simulink model "mstruct_bus1"  (Simulink 6.3)
settings: Solver=ode5  StartTime=0.0  StopTime=30  RelTol=1e-3
PreLoadFcn:
  | load mstruct_bus1_data
settings Model: Creator=The MathWorks Inc.  LastModifiedBy=mshakeri  ExtModeAutoUpdateStatusClock=off  StrictBusMsg=ErrorLevel1
settings DataIOCC: SignalLoggingName=logsOut
settings OptimizationCC: InlineParams=on  InlineInvariantSignals=on
settings DebuggingCC: CheckExecutionContextPreStartOutputMsg=on  CheckExecutionContextRuntimeOutputMsg=on  SolverPrmCheckMsg=none
settings HardwareCC: TargetHWDeviceType=32-bit Generic
settings ModelReferenceCC: UpdateModelReferenceTargets=IfOutOfDate
settings RTWCC: ProcessScript=grt_make_rtw_hook

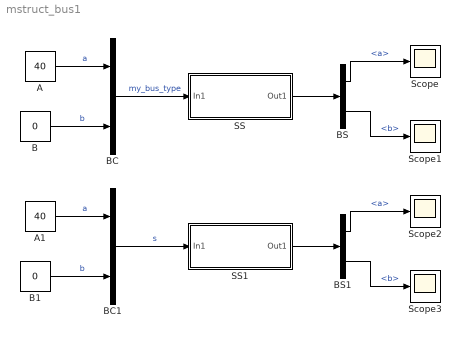
== system mstruct_bus1 ==
  A : Constant  Value=40  OutDataTypeMode=double  SampleTime=0.1
  A1 : Constant  Value=40  OutDataTypeMode=double  SampleTime=0.1
  B : Constant  Value=0  OutDataTypeMode=double  SampleTime=0.1
  B1 : Constant  Value=0  OutDataTypeMode=double  SampleTime=0.1
  BC : BusCreator  Inputs=2  NonVirtualBus=on
  BC1 : BusCreator  Inputs=2  UseBusObject=on  NonVirtualBus=on
      settings: BusObject=BC
  BS : BusSelector  OutputSignals=a,b
  BS1 : BusSelector  OutputSignals=a,b
  SS : Subsystem  TreatAsAtomicUnit=on
  SS1 : Subsystem  TreatAsAtomicUnit=on
  Scope{,1..3} (4 alike) : Scope
      Scope settings: TimeRange=30  YMax=50  DataFormat=Array
      Scope1 settings: TimeRange=30  YMax=50  DataFormat=Array
      Scope2 settings: TimeRange=30  YMax=50  SaveName=ScopeData2  DataFormat=Array
      Scope3 settings: TimeRange=30  YMax=50  SaveName=ScopeData3  DataFormat=Array
  wires:
  A/1 -> BC/1  "a"
  B/1 -> BC/2  "b"
  BC/1 -> SS/1(In1)  "my_bus_type"
  SS/1(Out1) -> BS/1
  BS/1 -> Scope/1  "<a>"
  BS/2 -> Scope1/1  "<b>"
  A1/1 -> BC1/1  "a"
  B1/1 -> BC1/2  "b"
  BC1/1 -> SS1/1(In1)  "s"
  SS1/1(Out1) -> BS1/1
  BS1/1 -> Scope2/1  "<a>"
  BS1/2 -> Scope3/1  "<b>"

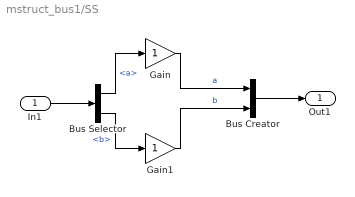
== system mstruct_bus1/SS ==
  In1 : Inport  Port=1  LatchInput=off
  Bus Creator : BusCreator  Inputs=2
  Bus Selector : BusSelector  OutputSignals=a,b
  Gain : Gain
  Gain1 : Gain
  Out1 : Outport
  wires:
  In1/1 -> Bus Selector/1
  Bus Selector/1 -> Gain/1  "<a>"
  Bus Selector/2 -> Gain1/1  "<b>"
  Gain/1 -> Bus Creator/1  "a"
  Gain1/1 -> Bus Creator/2  "b"
  Bus Creator/1 -> Out1/1

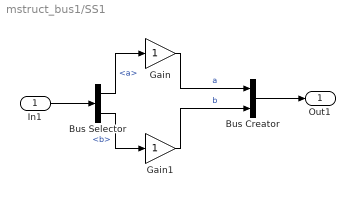
== system mstruct_bus1/SS1 ==
  In1 : Inport  Port=1  LatchInput=off
  Bus Creator : BusCreator  Inputs=2  UseBusObject=on  NonVirtualBus=on
      settings: BusObject=BC
  Bus Selector : BusSelector  OutputSignals=a,b
  Gain : Gain
  Gain1 : Gain
  Out1 : Outport
  wires:
  Bus Creator/1 -> Out1/1
  Gain1/1 -> Bus Creator/2  "b"
  Gain/1 -> Bus Creator/1  "a"
  Bus Selector/2 -> Gain1/1  "<b>"
  Bus Selector/1 -> Gain/1  "<a>"
  In1/1 -> Bus Selector/1
